simulink model "lv_demo5"  (Simulink 7.1)
settings: Solver=ode45  StartTime=0.0  StopTime=12  FixedStep=0.01  RelTol=1e-3
values from neighbouring files (symbols this model uses):
  C1 = 0.44    [lv_demofile.m]    (also in lv_demofile1.m; lv_demofile2.m; lv_demofile4.m; lv_demofile5.m)
  C2 = 0.0167    [lv_demofile.m]    (also in lv_demofile1.m; lv_demofile2.m; lv_demofile4.m; lv_demofile5.m)
  C3 = 0.3    [lv_demofile.m]    (also in lv_demofile1.m; lv_demofile2.m; lv_demofile4.m; lv_demofile5.m)
  C4 = 0.00184    [lv_demofile.m]    (also in lv_demofile1.m; lv_demofile2.m; lv_demofile4.m; lv_demofile5.m)
  cut_in = 3    [lv_cankaofile.m]    (also in lv_demofile.m; lv_demofile1.m; lv_demofile2.m; lv_demofile3.m)
  cut_out = 25    [lv_cankaofile.m]    (also in lv_demofile.m; lv_demofile1.m; lv_demofile2.m; lv_demofile3.m)
  Jem = 90    [lv_cankaofile.m]    (also in lv_demofile.m = 97.5; lv_demofile1.m = 97.5; lv_demofile2.m = 97.5; lv_demofile3.m = 97.5)
  Jwt = 9e7    (= 90000000)    [lv_cankaofile.m]    (also in lv_demofile.m = 3275300; lv_demofile1.m = 3275300; lv_demofile2.m = 3275300; lv_demofile3.m = 3275300)
  K = 83    [lv_cankaofile.m]    (also in lv_demofile.m; lv_demofile1.m = 75.76; lv_demofile2.m; lv_demofile3.m = 75.76)
  R = 40    [lv_cankaofile.m]    (also in lv_demofile.m = 38.5; lv_demofile1.m = 38.75; lv_demofile2.m = 38.5; lv_demofile3.m = 38.5)
  ro_air = 1.225    [lv_cankaofile.m]    (also in lv_demofile.m = 1.2236; lv_demofile1.m; lv_demofile2.m = 1.2236; lv_demofile3.m)
  Tact = 0    [lv_cankaofile.m]    (also in lv_demofile.m; lv_demofile1.m; lv_demofile2.m; lv_demofile3.m)
libraries: wt_blockset_v3 x1
settings Model: Creator=lv  LastModifiedBy=lv

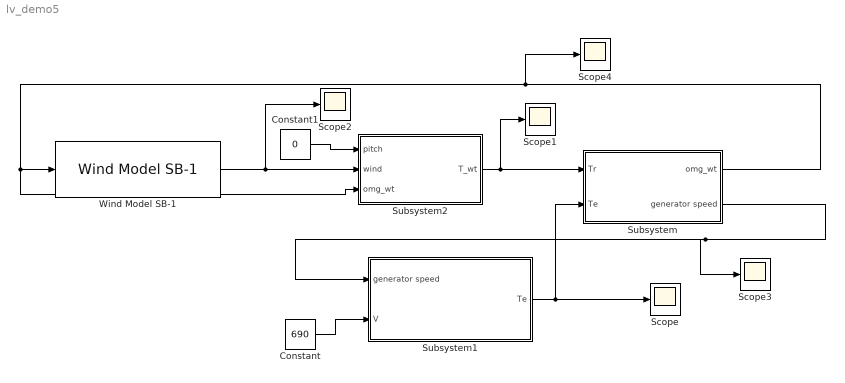
== system lv_demo5 ==
  Constant : Constant  Value=690  OutDataType=sfix(16)  OutScaling=2^0
  Constant1 : Constant  Value=0  OutDataType=sfix(16)  OutScaling=2^0
  Scope{,1..4} (5 alike) : Scope
      Scope1 settings: TimeRange=12  YMin=250000  YMax=550000  SaveName=ScopeData2
      Scope2 settings: SaveName=ScopeData3
      Scope3 settings: SaveName=ScopeData4
      Scope4 settings: TimeRange=12  YMin=-2  YMax=0  SaveName=ScopeData5
  Subsystem : Subsystem
  Subsystem1 : Subsystem
  Subsystem2 : Subsystem
  Wind Model SB-1 : wt_blockset_v3/Mechanical Components/Wind Model SB-1  SystemSampleTime=-1  D_rotor=72  v_mean=10  roughness=600  turb_int=12  T_sample=0.05
  wires:
  Subsystem2/1(T_wt) -> Scope1/1, Subsystem/1(Tr)
  Subsystem/2(generator speed) -> Scope3/1, Subsystem1/1(generator speed)
  Subsystem1/1(Te) -> Scope/1, Subsystem/2(Te)
  Subsystem/1(omg_wt) -> Scope4/1, Subsystem2/3(omg_wt), Wind Model SB-1/1
  Wind Model SB-1/1 -> Scope2/1, Subsystem2/2(wind)
  Constant/1 -> Subsystem1/2(V)
  Constant1/1 -> Subsystem2/1(pitch)

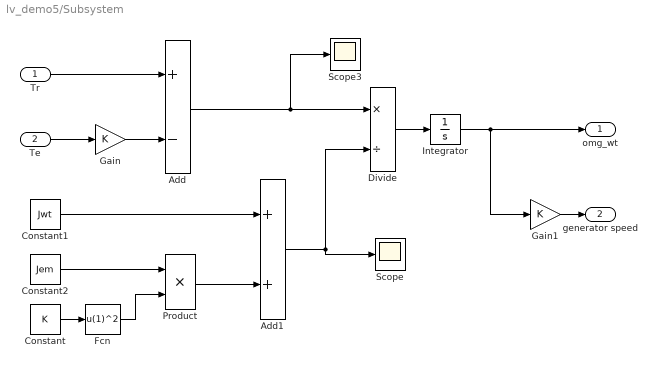
== system lv_demo5/Subsystem ==
  Tr : Inport  OutDataType=sfix(16)  OutScaling=2^0
  Te : Inport  Port=2  OutDataType=sfix(16)  OutScaling=2^0
  Add : Sum  Inputs=+-  OutDataType=sfix(16)  OutScaling=2^-10
  Add1 : Sum  OutDataType=sfix(16)  OutScaling=2^-10
  Constant : Constant  Value=K  OutDataType=sfix(16)  OutScaling=2^0
  Constant1 : Constant  Value=Jwt  OutDataType=sfix(16)  OutScaling=2^0
  Constant2 : Constant  Value=Jem  OutDataType=sfix(16)  OutScaling=2^0
  Divide : Product  Inputs=*/  OutDataType=sfix(16)  OutScaling=2^-10
  Fcn : Fcn  Expr=u(1)^2
  Gain : Gain  Gain=K  ParameterDataType=sfix(16)  ParameterScaling=2^0  OutDataType=sfix(16)  OutScaling=2^0
  Gain1 : Gain  Gain=K  ParameterDataType=sfix(16)  ParameterScaling=2^0  OutDataType=sfix(16)  OutScaling=2^0
  Integrator : Integrator
  Product : Product  OutDataType=sfix(16)  OutScaling=2^0  RndMeth=Zero
  Scope : Scope
      settings: SaveName=ScopeData13
  Scope3 : Scope
      settings: SaveName=ScopeData9
  omg_wt : Outport  OutDataType=sfix(16)  OutScaling=2^0
  generator speed : Outport  Port=2  OutDataType=sfix(16)  OutScaling=2^0
  wires:
  Gain1/1 -> generator speed/1
  Add1/1 -> Divide/2, Scope/1
  Add/1 -> Divide/1, Scope3/1
  Product/1 -> Add1/2
  Constant1/1 -> Add1/1
  Constant2/1 -> Product/1
  Gain/1 -> Add/2
  Tr/1 -> Add/1
  Te/1 -> Gain/1
  Constant/1 -> Fcn/1
  Fcn/1 -> Product/2
  Divide/1 -> Integrator/1
  Integrator/1 -> omg_wt/1, Gain1/1

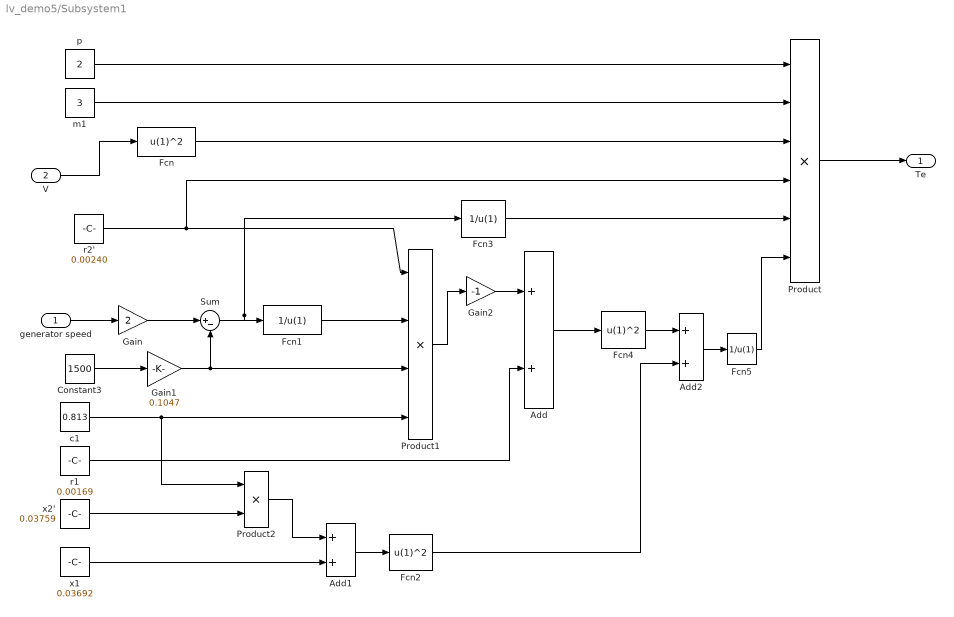
== system lv_demo5/Subsystem1 ==
  generator speed : Inport  OutDataType=sfix(16)  OutScaling=2^0
  V : Inport  Port=2  OutDataType=sfix(16)  OutScaling=2^0
  Add : Sum  OutDataType=sfix(16)  OutScaling=2^-10
  Add1 : Sum  OutDataType=sfix(16)  OutScaling=2^-10
  Add2 : Sum  OutDataType=sfix(16)  OutScaling=2^-10
  Constant3 : Constant  Value=1500  OutDataType=sfix(16)  OutScaling=2^0
  Fcn : Fcn  Expr=u(1)^2
  Fcn1 : Fcn  Expr=1/u(1)
  Fcn2 : Fcn  Expr=u(1)^2
  Fcn3 : Fcn  Expr=1/u(1)
  Fcn4 : Fcn  Expr=u(1)^2
  Fcn5 : Fcn  Expr=1/u(1)
  Gain : Gain  Gain=2  ParameterDataType=sfix(16)  ParameterScaling=2^0  OutDataType=sfix(16)  OutScaling=2^0
  Gain1 : Gain  Gain=0.1047  ParameterDataType=sfix(16)  ParameterScaling=2^0  OutDataType=sfix(16)  OutScaling=2^0
  Gain2 : Gain  Gain=-1  ParameterDataType=sfix(16)  ParameterScaling=2^0  OutDataType=sfix(16)  OutScaling=2^0
  Product : Product  Inputs=6  OutDataType=sfix(16)  OutScaling=2^0  RndMeth=Zero
  Product1 : Product  Inputs=4  OutDataType=sfix(16)  OutScaling=2^0  RndMeth=Zero
  Product2 : Product  OutDataType=sfix(16)  OutScaling=2^0  RndMeth=Zero
  Sum : Sum  Inputs=|+-  OutDataType=sfix(16)  OutScaling=2^0
  c1 : Constant  Value=0.813  OutDataType=sfix(16)  OutScaling=2^0
  m1 : Constant  Value=3  OutDataType=sfix(16)  OutScaling=2^0
  p : Constant  Value=2  OutDataType=sfix(16)  OutScaling=2^0
  r1 : Constant  Value=0.00169  OutDataType=sfix(16)  OutScaling=2^0
  r2' : Constant  Value=0.00240  OutDataType=sfix(16)  OutScaling=2^0
  x1 : Constant  Value=0.03692  OutDataType=sfix(16)  OutScaling=2^0
  x2' : Constant  Value=0.03759  OutDataType=sfix(16)  OutScaling=2^0
  Te : Outport  OutDataType=sfix(16)  OutScaling=2^0
  wires:
  V/1 -> Fcn/1
  generator speed/1 -> Gain/1
  Gain/1 -> Sum/1
  Constant3/1 -> Gain1/1
  Gain1/1 -> Sum/2, Product1/3
  Sum/1 -> Fcn3/1, Fcn1/1
  r2'/1 -> Product1/1, Product/4
  c1/1 -> Product1/4, Product2/1
  x2'/1 -> Product2/2
  Product2/1 -> Add1/1
  x1/1 -> Add1/2
  Add1/1 -> Fcn2/1
  Product1/1 -> Gain2/1
  p/1 -> Product/1
  m1/1 -> Product/2
  Fcn/1 -> Product/3
  r1/1 -> Add/2
  Gain2/1 -> Add/1
  Fcn3/1 -> Product/5
  Add/1 -> Fcn4/1
  Fcn4/1 -> Add2/1
  Fcn2/1 -> Add2/2
  Add2/1 -> Fcn5/1
  Fcn5/1 -> Product/6
  Product/1 -> Te/1
  Fcn1/1 -> Product1/2

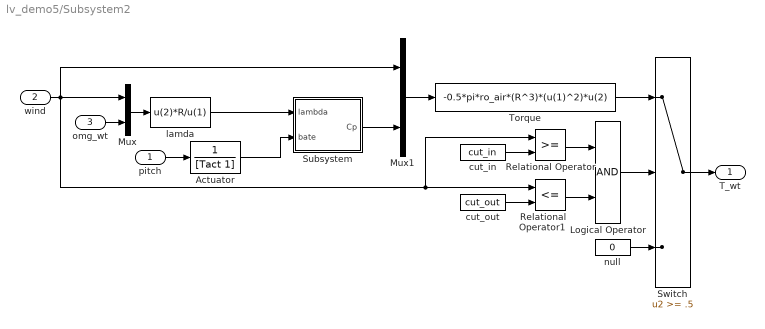
== system lv_demo5/Subsystem2 ==
  pitch : Inport  OutDataType=sfix(16)  OutScaling=2^0
  wind : Inport  Port=2  OutDataType=sfix(16)  OutScaling=2^0
  omg_wt : Inport  Port=3  OutDataType=sfix(16)  OutScaling=2^0
  Actuator : TransferFcn  Denominator=[Tact 1]
  Logical Operator : Logic
  Mux : Mux  Inputs=2
  Mux1 : Mux  Inputs=2
  Relational Operator : RelationalOperator  InputSameDT=on
  Relational Operator1 : RelationalOperator  Operator=<=  InputSameDT=on
  Subsystem : Subsystem
  Switch : Switch  Threshold=.5  SaturateOnIntegerOverflow=on  InputSameDT=on
  Torque : Fcn  Expr=-0.5*pi*ro_air*(R^3)*(u(1)^2)*u(2)
  cut_in : Constant  Value=cut_in  OutDataType=sfix(16)  OutScaling=2^0
  cut_out : Constant  Value=cut_out  OutDataType=sfix(16)  OutScaling=2^0
  lamda : Fcn  Expr=u(2)*R/u(1)
  null : Constant  Value=0  OutDataType=sfix(16)  OutScaling=2^0
  T_wt : Outport  OutDataType=sfix(16)  OutScaling=2^0
  wires:
  pitch/1 -> Actuator/1
  lamda/1 -> Subsystem/1(lambda)
  Subsystem/1(Cp) -> Mux1/2
  wind/1 -> Mux1/1, Relational Operator1/1, Relational Operator/1, Mux/1
  Logical Operator/1 -> Switch/2
  null/1 -> Switch/3
  Torque/1 -> Switch/1
  Switch/1 -> T_wt/1
  Relational Operator/1 -> Logical Operator/1
  Relational Operator1/1 -> Logical Operator/2
  cut_out/1 -> Relational Operator1/2
  cut_in/1 -> Relational Operator/2
  omg_wt/1 -> Mux/2
  Mux1/1 -> Torque/1
  Mux/1 -> lamda/1
  Actuator/1 -> Subsystem/2(bate)

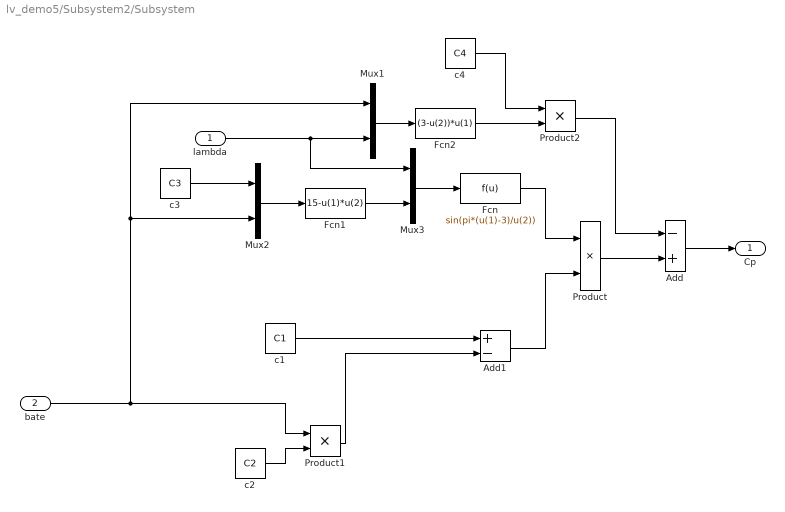
== system lv_demo5/Subsystem2/Subsystem ==
  lambda : Inport  OutDataType=sfix(16)  OutScaling=2^0
  bate : Inport  Port=2  OutDataType=sfix(16)  OutScaling=2^0
  Add : Sum  Inputs=-+  OutDataType=sfix(16)  OutScaling=2^-10
  Add1 : Sum  Inputs=+-  OutDataType=sfix(16)  OutScaling=2^-10
  Fcn : Fcn  Expr=sin(pi*(u(1)-3)/u(2))
  Fcn1 : Fcn  Expr=15-u(1)*u(2)
  Fcn2 : Fcn  Expr=(3-u(2))*u(1)
  Mux1 : Mux  Inputs=2
  Mux2 : Mux  Inputs=2
  Mux3 : Mux  Inputs=2
  Product : Product  OutDataType=sfix(16)  OutScaling=2^0  RndMeth=Zero
  Product1 : Product  OutDataType=sfix(16)  OutScaling=2^0  RndMeth=Zero
  Product2 : Product  OutDataType=sfix(16)  OutScaling=2^0  RndMeth=Zero
  c1 : Constant  Value=C1  OutDataType=sfix(16)  OutScaling=2^0
  c2 : Constant  Value=C2  OutDataType=sfix(16)  OutScaling=2^0
  c3 : Constant  Value=C3  OutDataType=sfix(16)  OutScaling=2^0
  c4 : Constant  Value=C4  OutDataType=sfix(16)  OutScaling=2^0
  Cp : Outport  OutDataType=sfix(16)  OutScaling=2^0
  wires:
  Add/1 -> Cp/1
  Product2/1 -> Add/1
  Fcn2/1 -> Product2/2
  c4/1 -> Product2/1
  Mux1/1 -> Fcn2/1
  lambda/1 -> Mux1/2, Mux3/1
  Fcn1/1 -> Mux3/2
  Product/1 -> Add/2
  Add1/1 -> Product/2
  Fcn/1 -> Product/1
  Mux3/1 -> Fcn/1
  c3/1 -> Mux2/1
  Mux2/1 -> Fcn1/1
  Product1/1 -> Add1/2
  c2/1 -> Product1/2
  bate/1 -> Mux1/1, Mux2/2, Product1/1
  c1/1 -> Add1/1
